simulink model "simulink_soft_ik"  (R2023b)
settings: Solver=ode15s  StartTime=0.0  StopTime=10.0  RelTol=1e-3
values from neighbouring files (symbols this model uses):
  L0 = 1    [class_test2D.m]    (also in class_test_hybrid.m = 0.5; test_bodyjacobian.m = 0.5; test_kinematics.m = 0.5; test_plot.m = 0.5)
  N_B = 1    [class_test2D.m]    (also in fd_mex_test.m = n; test_bodyjacobian.m = 2; test_kinematics.m = 2; test_plot.m)
  q_test = 1    [class_test2D.m]    (also in class_test_hybrid.m = [1; 1; 0.1; -1; 1; 0]; test_bodyjacobian.m = ones(r1.n, 1); test_kinematics.m = (q_max-q_min).*rand(r1.n,1) + q_min; test_plot.m = q_lb + (q_ub-q_lb).*rand(sr.n,1))
  r1 = BodyTree(J, B)    [class_test_hybrid.m]    (also in fd_mex_test.m = BodyTree(J1, B1); methods_test.m = BodyTree(J1, B1); test_bodyjacobian.m = BodyTree(J1, B1); test_kinematics.m = BodyTree(J1, B1))
  T = r1.DirectKinematics(q_test)    [test_kinematics.m]    (also in test_soft_kinematics.m = r1.DirectKinematics(q_test, L0*(1:N_B)))
libraries: SoftRobotics x1
settings Model: Creator=pietro  LastModifiedBy=pietro
settings RTWCC: GenerateReport=on

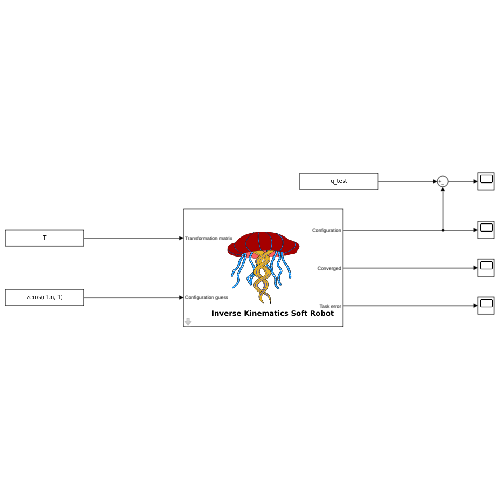
[thumbnail: Simulink's stored preview of the top-level diagram]
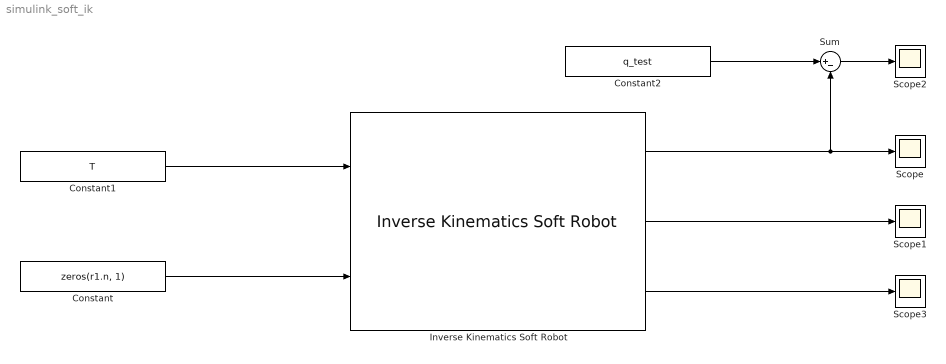
== system simulink_soft_ik ==
  Constant : Constant  Value=zeros(r1.n, 1)
  Constant1 : Constant  Value=T
  Constant2 : Constant  Value=q_test
  Inverse Kinematics Soft Robot : SoftRobotics/Inverse Kinematics Soft Robot  robotModel=r1  SimulateUsing=Code generation  BodyPoints=L0*(1:N_B)  MaximumNewtonIterations=200  TaskSpaceFlags=ones( 6*N_B, 1 )  AngularErrorThreshold=1e-3  LinearErrorThreshold=1e-2  UseGradientDescent=off  GradientDescentStepSize=0.2  ErrorWeight=1
      settings: SourceProductName=Jelly
  Scope{,1..3} (4 alike) : Scope
  Sum : Sum  Inputs=|+-
  wires:
  Constant/1 -> Inverse Kinematics Soft Robot/2
  Constant1/1 -> Inverse Kinematics Soft Robot/1
  Inverse Kinematics Soft Robot/1 -> Scope/1, Sum/2
  Inverse Kinematics Soft Robot/2 -> Scope1/1
  Sum/1 -> Scope2/1
  Constant2/1 -> Sum/1
  Inverse Kinematics Soft Robot/3 -> Scope3/1
